simulink model "wheel_leg_robot"  (R2023b)
settings: Solver=ode45  StartTime=0.0  StopTime=10  RelTol=1e-3  AbsTol=1e-3  EnableMultiTasking=on
values from neighbouring files (symbols this model uses):
  N = Nm + mp * (dd_x + L * dd_theta * cos(theta) - L * d_theta^2 * sin(theta))    [model.m]
undefined symbols (not defined in the file or in its folder): X, Y, Z
libraries: sm_lib x57, nesl_utility x19, slpidlib x5, simulink x1
(part 3 of 3)

== matlab function wheel_leg_robot/wheel_leg/MATLAB Function1 ==
  data: phi_1 input; d_phi_1 input; phi_4 input; L0_R output; phi0_R output; d_phi_4 input; d_phi0_R output
function [L0_R, phi0_R, d_phi0_R] = fcn(phi_1, d_phi_1, phi_4, d_phi_4)

    l1 = 0.15;
    l2 = 0.27;
    l3 = l2;
    l4 = l1;
    l5 = 0.15;
    Xb = l1 * cos(phi_1);
    Yb = l1 * sin(phi_1);
    Xd = l4 * cos(phi_4) + l5;
    Yd = l4 * sin(phi_4);
    lbd = sqrt((Xd - Xb)^2 + (Yd - Yb)^2);
    A0 = 2 * l2 * (Xd - Xb);
    B0 = 2 * l2 * (Yd - Yb);
    C0 = l2^2 + lbd^2 - l3^2;
    phi_2 = 2 * atan2((B0 + sqrt(A0^2 + B0^2 - C0^2)), (A0 + C0));
    Xc = Xb + l2 * cos(phi_2);
    Yc = Yb + l2 * sin(phi_2);

    L0_R = sqrt((Xc - l5/2)^2 + Yc^2);
    phi0_R = atan2(Yc, (Xc - l5/2));

    d_phi0_R = (d_phi_1*((l1*cos(phi_1) + (2*l2*cos(2*atan(((4*l2^2*(l1*sin(phi_1) - l4*sin(phi_4))^2 - ((l1*sin(phi_1) - l4*sin(phi_4))^2 + (l5 - l1*cos(phi_1) + l4*cos(phi_4))^2 + l2^2 - l3^2)^2 + 4*l2^2*(l5 - l1*cos(phi_1) + l4*cos(phi_4))^2)^(1/2) - 2*l2*(l1*sin(phi_1) - l4*sin(phi_4)))/((l1*sin(phi_1) - l4*sin(phi_4))^2 + (l5 - l1*cos(phi_1) + l4*cos(phi_4))^2 + l2^2 - l3^2 + 2*l2*(l5 - l1*cos(phi_1) + l4*cos(phi_4)))))*(((8*l1*l2^2*cos(phi_1)*(l1*sin(phi_1) - l4*sin(phi_4)) - 2*(2*l1*cos(phi_1)*(l1*sin(phi_1) - l4*sin(phi_4)) + 2*l1*sin(phi_1)*(l5 - l1*cos(phi_1) + l4*cos(phi_4)))*((l1*sin(phi_1) - l4*sin(phi_4))^2 + (l5 - l1*cos(phi_1) + l4*cos(phi_4))^2 + l2^2 - l3^2) + 8*l1*l2^2*sin(phi_1)*(l5 - l1*cos(phi_1) + l4*cos(phi_4)))/(2*(4*l2^2*(l1*sin(phi_1) - l4*sin(phi_4))^2 - ((l1*sin(phi_1) - l4*sin(phi_4))^2 + (l5 - l1*cos(phi_1) + l4*cos(phi_4))^2 + l2^2 - l3^2)^2 + 4*l2^2*(l5 - l1*cos(phi_1) + l4*cos(phi_4))^2)^(1/2)) - 2*l1*l2*cos(phi_1))/((l1*sin(phi_1) - l4*sin(phi_4))^2 + (l5 - l1*cos(phi_1) + l4*cos(phi_4))^2 + l2^2 - l3^2 + 2*l2*(l5 - l1*cos(phi_1) + l4*cos(phi_4))) - (((4*l2^2*(l1*sin(phi_1) - l4*sin(phi_4))^2 - ((l1*sin(phi_1) - l4*sin(phi_4))^2 + (l5 - l1*cos(phi_1) + l4*cos(phi_4))^2 + l2^2 - l3^2)^2 + 4*l2^2*(l5 - l1*cos(phi_1) + l4*cos(phi_4))^2)^(1/2) - 2*l2*(l1*sin(phi_1) - l4*sin(phi_4)))*(2*l1*l2*sin(phi_1) + 2*l1*cos(phi_1)*(l1*sin(phi_1) - l4*sin(phi_4)) + 2*l1*sin(phi_1)*(l5 - l1*cos(phi_1) + l4*cos(phi_4))))/((l1*sin(phi_1) - l4*sin(phi_4))^2 + (l5 - l1*cos(phi_1) + l4*cos(phi_4))^2 + l2^2 - l3^2 + 2*l2*(l5 - l1*cos(phi_1) + l4*cos(phi_4)))^2))/(((4*l2^2*(l1*sin(phi_1) - l4*sin(phi_4))^2 - ((l1*sin(phi_1) - l4*sin(phi_4))^2 + (l5 - l1*cos(phi_1) + l4*cos(phi_4))^2 + l2^2 - l3^2)^2 + 4*l2^2*(l5 - l1*cos(phi_1) + l4*cos(phi_4))^2)^(1/2) - 2*l2*(l1*sin(phi_1) - l4*sin(phi_4)))^2/((l1*sin(phi_1) - l4*sin(phi_4))^2 + (l5 - l1*cos(phi_1) + l4*cos(phi_4))^2 + l2^2 - l3^2 + 2*l2*(l5 - l1*cos(phi_1) + l4*cos(phi_4)))^2 + 1))/(l2*cos(2*atan(((4*l2^2*(l1*sin(phi_1) - l4*sin(phi_4))^2 - ((l1*sin(phi_1) - l4*sin(phi_4))^2 + (l5 - l1*cos(phi_1) + l4*cos(phi_4))^2 + l2^2 - l3^2)^2 + 4*l2^2*(l5 - l1*cos(phi_1) + l4*cos(phi_4))^2)^(1/2) - 2*l2*(l1*sin(phi_1) - l4*sin(phi_4)))/((l1*sin(phi_1) - l4*sin(phi_4))^2 + (l5 - l1*cos(phi_1) + l4*cos(phi_4))^2 + l2^2 - l3^2 + 2*l2*(l5 - l1*cos(phi_1) + l4*cos(phi_4))))) - l5/2 + l1*cos(phi_1)) + ((l2*sin(2*atan(((4*l2^2*(l1*sin(phi_1) - l4*sin(phi_4))^2 - ((l1*sin(phi_1) - l4*sin(phi_4))^2 + (l5 - l1*cos(phi_1) + l4*cos(phi_4))^2 + l2^2 - l3^2)^2 + 4*l2^2*(l5 - l1*cos(phi_1) + l4*cos(phi_4))^2)^(1/2) - 2*l2*(l1*sin(phi_1) - l4*sin(phi_4)))/((l1*sin(phi_1) - l4*sin(phi_4))^2 + (l5 - l1*cos(phi_1) + l4*cos(phi_4))^2 + l2^2 - l3^2 + 2*l2*(l5 - l1*cos(phi_1) + l4*cos(phi_4))))) + l1*sin(phi_1))*(l1*sin(phi_1) + (2*l2*sin(2*atan(((4*l2^2*(l1*sin(phi_1) - l4*sin(phi_4))^2 - ((l1*sin(phi_1) - l4*sin(phi_4))^2 + (l5 - l1*cos(phi_1) + l4*cos(phi_4))^2 + l2^2 - l3^2)^2 + 4*l2^2*(l5 - l1*cos(phi_1) + l4*cos(phi_4))^2)^(1/2) - 2*l2*(l1*sin(phi_1) - l4*sin(phi_4)))/((l1*sin(phi_1) - l4*sin(phi_4))^2 + (l5 - l1*cos(phi_1) + l4*cos(phi_4))^2 + l2^2 - l3^2 + 2*l2*(l5 - l1*cos(phi_1) + l4*cos(phi_4)))))*(((8*l1*l2^2*cos(phi_1)*(l1*sin(phi_1) - l4*sin(phi_4)) - 2*(2*l1*cos(phi_1)*(l1*sin(phi_1) - l4*sin(phi_4)) + 2*l1*sin(phi_1)*(l5 - l1*cos(phi_1) + l4*cos(phi_4)))*((l1*sin(phi_1) - l4*sin(phi_4))^2 + (l5 - l1*cos(phi_1) + l4*cos(phi_4))^2 + l2^2 - l3^2) + 8*l1*l2^2*sin(phi_1)*(l5 - l1*cos(phi_1) + l4*cos(phi_4)))/(2*(4*l2^2*(l1*sin(phi_1) - l4*sin(phi_4))^2 - ((l1*sin(phi_1) - l4*sin(phi_4))^2 + (l5 - l1*cos(phi_1) + l4*cos(phi_4))^2 + l2^2 - l3^2)^2 + 4*l2^2*(l5 - l1*cos(phi_1) + l4*cos(phi_4))^2)^(1/2)) - 2*l1*l2*cos(phi_1))/((l1*sin(phi_1) - l4*sin(phi_4))^2 + (l5 - l1*cos(phi_1) + l4*cos(phi_4))^2 + l2^2 - l3^2 + 2*l2*(l5 - l1*cos(phi_1) + l4*cos(phi_4))) - (((4*l2^2*(l1*sin(phi_1) - l4*sin(phi_4))^2 - ((l1*sin(phi_1) - l4*sin(phi_4))^2 + (l5 - l1*cos(phi_1) + l4*cos(phi_4))^2 + l2^2 - l3^2)^2 + 4*l2^2*(l5 - l1*cos(phi_1) + l4*cos(phi_4))^2)^(1/2) - 2*l2*(l1*sin(phi_1) - l4*sin(phi_4)))*(2*l1*l2*sin(phi_1) + 2*l1*cos(phi_1)*(l1*sin(phi_1) - l4*sin(phi_4)) + 2*l1*sin(phi_1)*(l5 - l1*cos(phi_1) + l4*cos(phi_4))))/((l1*sin(phi_1) - l4*sin(phi_4))^2 + (l5 - l1*cos(phi_1) + l4*cos(phi_4))^2 + l2^2 - l3^2 + 2*l2*(l5 - l1*cos(phi_1) + l4*cos(phi_4)))^2))/(((4*l2^2*(l1*sin(phi_1) - l4*sin(phi_4))^2 - ((l1*sin(phi_1) - l4*sin(phi_4))^2 + (l5 - l1*cos(phi_1) + l4*cos(phi_4))^2 + l2^2 - l3^2)^2 + 4*l2^2*(l5 - l1*cos(phi_1) + l4*cos(phi_4))^2)^(1/2) - 2*l2*(l1*sin(phi_1) - l4*sin(phi_4)))^2/((l1*sin(phi_1) - l4*sin(phi_4))^2 + (l5 - l1*cos(phi_1) + l4*cos(phi_4))^2 + l2^2 - l3^2 + 2*l2*(l5 - l1*cos(phi_1) + l4*cos(phi_4)))^2 + 1)))/(l2*cos(2*atan(((4*l2^2*(l1*sin(phi_1) - l4*sin(phi_4))^2 - ((l1*sin(phi_1) - l4*sin(phi_4))^2 + (l5 - l1*cos(phi_1) + l4*cos(phi_4))^2 + l2^2 - l3^2)^2 + 4*l2^2*(l5 - l1*cos(phi_1) + l4*cos(phi_4))^2)^(1/2) - 2*l2*(l1*sin(phi_1) - l4*sin(phi_4)))/((l1*sin(phi_1) - l4*sin(phi_4))^2 + (l5 - l1*cos(phi_1) + l4*cos(phi_4))^2 + l2^2 - l3^2 + 2*l2*(l5 - l1*cos(phi_1) + l4*cos(phi_4))))) - l5/2 + l1*cos(phi_1))^2))/((l2*sin(2*atan(((4*l2^2*(l1*sin(phi_1) - l4*sin(phi_4))^2 - ((l1*sin(phi_1) - l4*sin(phi_4))^2 + (l5 - l1*cos(phi_1) + l4*cos(phi_4))^2 + l2^2 - l3^2)^2 + 4*l2^2*(l5 - l1*cos(phi_1) + l4*cos(phi_4))^2)^(1/2) - 2*l2*(l1*sin(phi_1) - l4*sin(phi_4)))/((l1*sin(phi_1) - l4*sin(phi_4))^2 + (l5 - l1*cos(phi_1) + l4*cos(phi_4))^2 + l2^2 - l3^2 + 2*l2*(l5 - l1*cos(phi_1) + l4*cos(phi_4))))) + l1*sin(phi_1))^2/(l2*cos(2*atan(((4*l2^2*(l1*sin(phi_1) - l4*sin(phi_4))^2 - ((l1*sin(phi_1) - l4*sin(phi_4))^2 + (l5 - l1*cos(phi_1) + l4*cos(phi_4))^2 + l2^2 - l3^2)^2 + 4*l2^2*(l5 - l1*cos(phi_1) + l4*cos(phi_4))^2)^(1/2) - 2*l2*(l1*sin(phi_1) - l4*sin(phi_4)))/((l1*sin(phi_1) - l4*sin(phi_4))^2 + (l5 - l1*cos(phi_1) + l4*cos(phi_4))^2 + l2^2 - l3^2 + 2*l2*(l5 - l1*cos(phi_1) + l4*cos(phi_4))))) - l5/2 + l1*cos(phi_1))^2 + 1) - (d_phi_4*((2*l2*cos(2*atan(((4*l2^2*(l1*sin(phi_1) - l4*sin(phi_4))^2 - ((l1*sin(phi_1) - l4*sin(phi_4))^2 + (l5 - l1*cos(phi_1) + l4*cos(phi_4))^2 + l2^2 - l3^2)^2 + 4*l2^2*(l5 - l1*cos(phi_1) + l4*cos(phi_4))^2)^(1/2) - 2*l2*(l1*sin(phi_1) - l4*sin(phi_4)))/((l1*sin(phi_1) - l4*sin(phi_4))^2 + (l5 - l1*cos(phi_1) + l4*cos(phi_4))^2 + l2^2 - l3^2 + 2*l2*(l5 - l1*cos(phi_1) + l4*cos(phi_4)))))*(((8*l2^2*l4*cos(phi_4)*(l1*sin(phi_1) - l4*sin(phi_4)) - 2*(2*l4*cos(phi_4)*(l1*sin(phi_1) - l4*sin(phi_4)) + 2*l4*sin(phi_4)*(l5 - l1*cos(phi_1) + l4*cos(phi_4)))*((l1*sin(phi_1) - l4*sin(phi_4))^2 + (l5 - l1*cos(phi_1) + l4*cos(phi_4))^2 + l2^2 - l3^2) + 8*l2^2*l4*sin(phi_4)*(l5 - l1*cos(phi_1) + l4*cos(phi_4)))/(2*(4*l2^2*(l1*sin(phi_1) - l4*sin(phi_4))^2 - ((l1*sin(phi_1) - l4*sin(phi_4))^2 + (l5 - l1*cos(phi_1) + l4*cos(phi_4))^2 + l2^2 - l3^2)^2 + 4*l2^2*(l5 - l1*cos(phi_1) + l4*cos(phi_4))^2)^(1/2)) - 2*l2*l4*cos(phi_4))/((l1*sin(phi_1) - l4*sin(phi_4))^2 + (l5 - l1*cos(phi_1) + l4*cos(phi_4))^2 + l2^2 - l3^2 + 2*l2*(l5 - l1*cos(phi_1) + l4*cos(phi_4))) - (((4*l2^2*(l1*sin(phi_1) - l4*sin(phi_4))^2 - ((l1*sin(phi_1) - l4*sin(phi_4))^2 + (l5 - l1*cos(phi_1) + l4*cos(phi_4))^2 + l2^2 - l3^2)^2 + 4*l2^2*(l5 - l1*cos(phi_1) + l4*cos(phi_4))^2)^(1/2) - 2*l2*(l1*sin(phi_1) - l4*sin(phi_4)))*(2*l2*l4*sin(phi_4) + 2*l4*cos(phi_4)*(l1*sin(phi_1) - l4*sin(phi_4)) + 2*l4*sin(phi_4)*(l5 - l1*cos(phi_1) + l4*cos(phi_4))))/((l1*sin(phi_1) - l4*sin(phi_4))^2 + (l5 - l1*cos(phi_1) + l4*cos(phi_4))^2 + l2^2 - l3^2 + 2*l2*(l5 - l1*cos(phi_1) + l4*cos(phi_4)))^2))/((((4*l2^2*(l1*sin(phi_1) - l4*sin(phi_4))^2 - ((l1*sin(phi_1) - l4*sin(phi_4))^2 + (l5 - l1*cos(phi_1) + l4*cos(phi_4))^2 + l2^2 - l3^2)^2 + 4*l2^2*(l5 - l1*cos(phi_1) + l4*cos(phi_4))^2)^(1/2) - 2*l2*(l1*sin(phi_1) - l4*sin(phi_4)))^2/((l1*sin(phi_1) - l4*sin(phi_4))^2 + (l5 - l1*cos(phi_1) + l4*cos(phi_4))^2 + l2^2 - l3^2 + 2*l2*(l5 - l1*cos(phi_1) + l4*cos(phi_4)))^2 + 1)*(l2*cos(2*atan(((4*l2^2*(l1*sin(phi_1) - l4*sin(phi_4))^2 - ((l1*sin(phi_1) - l4*sin(phi_4))^2 + (l5 - l1*cos(phi_1) + l4*cos(phi_4))^2 + l2^2 - l3^2)^2 + 4*l2^2*(l5 - l1*cos(phi_1) + l4*cos(phi_4))^2)^(1/2) - 2*l2*(l1*sin(phi_1) - l4*sin(phi_4)))/((l1*sin(phi_1) - l4*sin(phi_4))^2 + (l5 - l1*cos(phi_1) + l4*cos(phi_4))^2 + l2^2 - l3^2 + 2*l2*(l5 - l1*cos(phi_1) + l4*cos(phi_4))))) - l5/2 + l1*cos(phi_1))) + (2*l2*sin(2*atan(((4*l2^2*(l1*sin(phi_1) - l4*sin(phi_4))^2 - ((l1*sin(phi_1) - l4*sin(phi_4))^2 + (l5 - l1*cos(phi_1) + l4*cos(phi_4))^2 + l2^2 - l3^2)^2 + 4*l2^2*(l5 - l1*cos(phi_1) + l4*cos(phi_4))^2)^(1/2) - 2*l2*(l1*sin(phi_1) - l4*sin(phi_4)))/((l1*sin(phi_1) - l4*sin(phi_4))^2 + (l5 - l1*cos(phi_1) + l4*cos(phi_4))^2 + l2^2 - l3^2 + 2*l2*(l5 - l1*cos(phi_1) + l4*cos(phi_4)))))*(l2*sin(2*atan(((4*l2^2*(l1*sin(phi_1) - l4*sin(phi_4))^2 - ((l1*sin(phi_1) - l4*sin(phi_4))^2 + (l5 - l1*cos(phi_1) + l4*cos(phi_4))^2 + l2^2 - l3^2)^2 + 4*l2^2*(l5 - l1*cos(phi_1) + l4*cos(phi_4))^2)^(1/2) - 2*l2*(l1*sin(phi_1) - l4*sin(phi_4)))/((l1*sin(phi_1) - l4*sin(phi_4))^2 + (l5 - l1*cos(phi_1) + l4*cos(phi_4))^2 + l2^2 - l3^2 + 2*l2*(l5 - l1*cos(phi_1) + l4*cos(phi_4))))) + l1*sin(phi_1))*(((8*l2^2*l4*cos(phi_4)*(l1*sin(phi_1) - l4*sin(phi_4)) - 2*(2*l4*cos(phi_4)*(l1*sin(phi_1) - l4*sin(phi_4)) + 2*l4*sin(phi_4)*(l5 - l1*cos(phi_1) + l4*cos(phi_4)))*((l1*sin(phi_1) - l4*sin(phi_4))^2 + (l5 - l1*cos(phi_1) + l4*cos(phi_4))^2 + l2^2 - l3^2) + 8*l2^2*l4*sin(phi_4)*(l5 - l1*cos(phi_1) + l4*cos(phi_4)))/(2*(4*l2^2*(l1*sin(phi_1) - l4*sin(phi_4))^2 - ((l1*sin(phi_1) - l4*sin(phi_4))^2 + (l5 - l1*cos(phi_1) + l4*cos(phi_4))^2 + l2^2 - l3^2)^2 + 4*l2^2*(l5 - l1*cos(phi_1) + l4*cos(phi_4))^2)^(1/2)) - 2*l2*l4*cos(phi_4))/((l1*sin(phi_1) - l4*sin(phi_4))^2 + (l5 - l1*cos(phi_1) + l4*cos(phi_4))^2 + l2^2 - l3^2 + 2*l2*(l5 - l1*cos(phi_1) + l4*cos(phi_4))) - (((4*l2^2*(l1*sin(phi_1) - l4*sin(phi_4))^2 - ((l1*sin(phi_1) - l4*sin(phi_4))^2 + (l5 - l1*cos(phi_1) + l4*cos(phi_4))^2 + l2^2 - l3^2)^2 + 4*l2^2*(l5 - l1*cos(phi_1) + l4*cos(phi_4))^2)^(1/2) - 2*l2*(l1*sin(phi_1) - l4*sin(phi_4)))*(2*l2*l4*sin(phi_4) + 2*l4*cos(phi_4)*(l1*sin(phi_1) - l4*sin(phi_4)) + 2*l4*sin(phi_4)*(l5 - l1*cos(phi_1) + l4*cos(phi_4))))/((l1*sin(phi_1) - l4*sin(phi_4))^2 + (l5 - l1*cos(phi_1) + l4*cos(phi_4))^2 + l2^2 - l3^2 + 2*l2*(l5 - l1*cos(phi_1) + l4*cos(phi_4)))^2))/((((4*l2^2*(l1*sin(phi_1) - l4*sin(phi_4))^2 - ((l1*sin(phi_1) - l4*sin(phi_4))^2 + (l5 - l1*cos(phi_1) + l4*cos(phi_4))^2 + l2^2 - l3^2)^2 + 4*l2^2*(l5 - l1*cos(phi_1) + l4*cos(phi_4))^2)^(1/2) - 2*l2*(l1*sin(phi_1) - l4*sin(phi_4)))^2/((l1*sin(phi_1) - l4*sin(phi_4))^2 + (l5 - l1*cos(phi_1) + l4*cos(phi_4))^2 + l2^2 - l3^2 + 2*l2*(l5 - l1*cos(phi_1) + l4*cos(phi_4)))^2 + 1)*(l2*cos(2*atan(((4*l2^2*(l1*sin(phi_1) - l4*sin(phi_4))^2 - ((l1*sin(phi_1) - l4*sin(phi_4))^2 + (l5 - l1*cos(phi_1) + l4*cos(phi_4))^2 + l2^2 - l3^2)^2 + 4*l2^2*(l5 - l1*cos(phi_1) + l4*cos(phi_4))^2)^(1/2) - 2*l2*(l1*sin(phi_1) - l4*sin(phi_4)))/((l1*sin(phi_1) - l4*sin(phi_4))^2 + (l5 - l1*cos(phi_1) + l4*cos(phi_4))^2 + l2^2 - l3^2 + 2*l2*(l5 - l1*cos(phi_1) + l4*cos(phi_4))))) - l5/2 + l1*cos(phi_1))^2)))/((l2*sin(2*atan(((4*l2^2*(l1*sin(phi_1) - l4*sin(phi_4))^2 - ((l1*sin(phi_1) - l4*sin(phi_4))^2 + (l5 - l1*cos(phi_1) + l4*cos(phi_4))^2 + l2^2 - l3^2)^2 + 4*l2^2*(l5 - l1*cos(phi_1) + l4*cos(phi_4))^2)^(1/2) - 2*l2*(l1*sin(phi_1) - l4*sin(phi_4)))/((l1*sin(phi_1) - l4*sin(phi_4))^2 + (l5 - l1*cos(phi_1) + l4*cos(phi_4))^2 + l2^2 - l3^2 + 2*l2*(l5 - l1*cos(phi_1) + l4*cos(phi_4))))) + l1*sin(phi_1))^2/(l2*cos(2*atan(((4*l2^2*(l1*sin(phi_1) - l4*sin(phi_4))^2 - ((l1*sin(phi_1) - l4*sin(phi_4))^2 + (l5 - l1*cos(phi_1) + l4*cos(phi_4))^2 + l2^2 - l3^2)^2 + 4*l2^2*(l5 - l1*cos(phi_1) + l4*cos(phi_4))^2)^(1/2) - 2*l2*(l1*sin(phi_1) - l4*sin(phi_4)))/((l1*sin(phi_1) - l4*sin(phi_4))^2 + (l5 - l1*cos(phi_1) + l4*cos(phi_4))^2 + l2^2 - l3^2 + 2*l2*(l5 - l1*cos(phi_1) + l4*cos(phi_4))))) - l5/2 + l1*cos(phi_1))^2 + 1);

== matlab function wheel_leg_robot/wheel_leg/MATLAB Function ==
  data: phi_1 input; d_phi_1 input; phi_4 input; L0_L output; phi0_L output; d_phi_4 input; d_phi0_L output
function [L0_L, phi0_L, d_phi0_L] = fcn(phi_1, d_phi_1, phi_4, d_phi_4)

    l1 = 0.15;
    l2 = 0.27;
    l3 = l2;
    l4 = l1;
    l5 = 0.15;
    Xb = l1 * cos(phi_1);
    Yb = l1 * sin(phi_1);
    Xd = l4 * cos(phi_4) + l5;
    Yd = l4 * sin(phi_4);
    lbd = sqrt((Xd - Xb)^2 + (Yd - Yb)^2);
    A0 = 2 * l2 * (Xd - Xb);
    B0 = 2 * l2 * (Yd - Yb);
    C0 = l2^2 + lbd^2 - l3^2;
    phi_2 = 2 * atan2((B0 + sqrt(A0^2 + B0^2 - C0^2)), (A0 + C0));
    Xc = Xb + l2 * cos(phi_2);
    Yc = Yb + l2 * sin(phi_2);

    L0_L = sqrt((Xc - l5/2)^2 + Yc^2);
    phi0_L = atan2(Yc, (Xc - l5/2));

    d_phi0_L = (d_phi_1*((l1*cos(phi_1) + (2*l2*cos(2*atan(((4*l2^2*(l1*sin(phi_1) - l4*sin(phi_4))^2 - ((l1*sin(phi_1) - l4*sin(phi_4))^2 + (l5 - l1*cos(phi_1) + l4*cos(phi_4))^2 + l2^2 - l3^2)^2 + 4*l2^2*(l5 - l1*cos(phi_1) + l4*cos(phi_4))^2)^(1/2) - 2*l2*(l1*sin(phi_1) - l4*sin(phi_4)))/((l1*sin(phi_1) - l4*sin(phi_4))^2 + (l5 - l1*cos(phi_1) + l4*cos(phi_4))^2 + l2^2 - l3^2 + 2*l2*(l5 - l1*cos(phi_1) + l4*cos(phi_4)))))*(((8*l1*l2^2*cos(phi_1)*(l1*sin(phi_1) - l4*sin(phi_4)) - 2*(2*l1*cos(phi_1)*(l1*sin(phi_1) - l4*sin(phi_4)) + 2*l1*sin(phi_1)*(l5 - l1*cos(phi_1) + l4*cos(phi_4)))*((l1*sin(phi_1) - l4*sin(phi_4))^2 + (l5 - l1*cos(phi_1) + l4*cos(phi_4))^2 + l2^2 - l3^2) + 8*l1*l2^2*sin(phi_1)*(l5 - l1*cos(phi_1) + l4*cos(phi_4)))/(2*(4*l2^2*(l1*sin(phi_1) - l4*sin(phi_4))^2 - ((l1*sin(phi_1) - l4*sin(phi_4))^2 + (l5 - l1*cos(phi_1) + l4*cos(phi_4))^2 + l2^2 - l3^2)^2 + 4*l2^2*(l5 - l1*cos(phi_1) + l4*cos(phi_4))^2)^(1/2)) - 2*l1*l2*cos(phi_1))/((l1*sin(phi_1) - l4*sin(phi_4))^2 + (l5 - l1*cos(phi_1) + l4*cos(phi_4))^2 + l2^2 - l3^2 + 2*l2*(l5 - l1*cos(phi_1) + l4*cos(phi_4))) - (((4*l2^2*(l1*sin(phi_1) - l4*sin(phi_4))^2 - ((l1*sin(phi_1) - l4*sin(phi_4))^2 + (l5 - l1*cos(phi_1) + l4*cos(phi_4))^2 + l2^2 - l3^2)^2 + 4*l2^2*(l5 - l1*cos(phi_1) + l4*cos(phi_4))^2)^(1/2) - 2*l2*(l1*sin(phi_1) - l4*sin(phi_4)))*(2*l1*l2*sin(phi_1) + 2*l1*cos(phi_1)*(l1*sin(phi_1) - l4*sin(phi_4)) + 2*l1*sin(phi_1)*(l5 - l1*cos(phi_1) + l4*cos(phi_4))))/((l1*sin(phi_1) - l4*sin(phi_4))^2 + (l5 - l1*cos(phi_1) + l4*cos(phi_4))^2 + l2^2 - l3^2 + 2*l2*(l5 - l1*cos(phi_1) + l4*cos(phi_4)))^2))/(((4*l2^2*(l1*sin(phi_1) - l4*sin(phi_4))^2 - ((l1*sin(phi_1) - l4*sin(phi_4))^2 + (l5 - l1*cos(phi_1) + l4*cos(phi_4))^2 + l2^2 - l3^2)^2 + 4*l2^2*(l5 - l1*cos(phi_1) + l4*cos(phi_4))^2)^(1/2) - 2*l2*(l1*sin(phi_1) - l4*sin(phi_4)))^2/((l1*sin(phi_1) - l4*sin(phi_4))^2 + (l5 - l1*cos(phi_1) + l4*cos(phi_4))^2 + l2^2 - l3^2 + 2*l2*(l5 - l1*cos(phi_1) + l4*cos(phi_4)))^2 + 1))/(l2*cos(2*atan(((4*l2^2*(l1*sin(phi_1) - l4*sin(phi_4))^2 - ((l1*sin(phi_1) - l4*sin(phi_4))^2 + (l5 - l1*cos(phi_1) + l4*cos(phi_4))^2 + l2^2 - l3^2)^2 + 4*l2^2*(l5 - l1*cos(phi_1) + l4*cos(phi_4))^2)^(1/2) - 2*l2*(l1*sin(phi_1) - l4*sin(phi_4)))/((l1*sin(phi_1) - l4*sin(phi_4))^2 + (l5 - l1*cos(phi_1) + l4*cos(phi_4))^2 + l2^2 - l3^2 + 2*l2*(l5 - l1*cos(phi_1) + l4*cos(phi_4))))) - l5/2 + l1*cos(phi_1)) + ((l2*sin(2*atan(((4*l2^2*(l1*sin(phi_1) - l4*sin(phi_4))^2 - ((l1*sin(phi_1) - l4*sin(phi_4))^2 + (l5 - l1*cos(phi_1) + l4*cos(phi_4))^2 + l2^2 - l3^2)^2 + 4*l2^2*(l5 - l1*cos(phi_1) + l4*cos(phi_4))^2)^(1/2) - 2*l2*(l1*sin(phi_1) - l4*sin(phi_4)))/((l1*sin(phi_1) - l4*sin(phi_4))^2 + (l5 - l1*cos(phi_1) + l4*cos(phi_4))^2 + l2^2 - l3^2 + 2*l2*(l5 - l1*cos(phi_1) + l4*cos(phi_4))))) + l1*sin(phi_1))*(l1*sin(phi_1) + (2*l2*sin(2*atan(((4*l2^2*(l1*sin(phi_1) - l4*sin(phi_4))^2 - ((l1*sin(phi_1) - l4*sin(phi_4))^2 + (l5 - l1*cos(phi_1) + l4*cos(phi_4))^2 + l2^2 - l3^2)^2 + 4*l2^2*(l5 - l1*cos(phi_1) + l4*cos(phi_4))^2)^(1/2) - 2*l2*(l1*sin(phi_1) - l4*sin(phi_4)))/((l1*sin(phi_1) - l4*sin(phi_4))^2 + (l5 - l1*cos(phi_1) + l4*cos(phi_4))^2 + l2^2 - l3^2 + 2*l2*(l5 - l1*cos(phi_1) + l4*cos(phi_4)))))*(((8*l1*l2^2*cos(phi_1)*(l1*sin(phi_1) - l4*sin(phi_4)) - 2*(2*l1*cos(phi_1)*(l1*sin(phi_1) - l4*sin(phi_4)) + 2*l1*sin(phi_1)*(l5 - l1*cos(phi_1) + l4*cos(phi_4)))*((l1*sin(phi_1) - l4*sin(phi_4))^2 + (l5 - l1*cos(phi_1) + l4*cos(phi_4))^2 + l2^2 - l3^2) + 8*l1*l2^2*sin(phi_1)*(l5 - l1*cos(phi_1) + l4*cos(phi_4)))/(2*(4*l2^2*(l1*sin(phi_1) - l4*sin(phi_4))^2 - ((l1*sin(phi_1) - l4*sin(phi_4))^2 + (l5 - l1*cos(phi_1) + l4*cos(phi_4))^2 + l2^2 - l3^2)^2 + 4*l2^2*(l5 - l1*cos(phi_1) + l4*cos(phi_4))^2)^(1/2)) - 2*l1*l2*cos(phi_1))/((l1*sin(phi_1) - l4*sin(phi_4))^2 + (l5 - l1*cos(phi_1) + l4*cos(phi_4))^2 + l2^2 - l3^2 + 2*l2*(l5 - l1*cos(phi_1) + l4*cos(phi_4))) - (((4*l2^2*(l1*sin(phi_1) - l4*sin(phi_4))^2 - ((l1*sin(phi_1) - l4*sin(phi_4))^2 + (l5 - l1*cos(phi_1) + l4*cos(phi_4))^2 + l2^2 - l3^2)^2 + 4*l2^2*(l5 - l1*cos(phi_1) + l4*cos(phi_4))^2)^(1/2) - 2*l2*(l1*sin(phi_1) - l4*sin(phi_4)))*(2*l1*l2*sin(phi_1) + 2*l1*cos(phi_1)*(l1*sin(phi_1) - l4*sin(phi_4)) + 2*l1*sin(phi_1)*(l5 - l1*cos(phi_1) + l4*cos(phi_4))))/((l1*sin(phi_1) - l4*sin(phi_4))^2 + (l5 - l1*cos(phi_1) + l4*cos(phi_4))^2 + l2^2 - l3^2 + 2*l2*(l5 - l1*cos(phi_1) + l4*cos(phi_4)))^2))/(((4*l2^2*(l1*sin(phi_1) - l4*sin(phi_4))^2 - ((l1*sin(phi_1) - l4*sin(phi_4))^2 + (l5 - l1*cos(phi_1) + l4*cos(phi_4))^2 + l2^2 - l3^2)^2 + 4*l2^2*(l5 - l1*cos(phi_1) + l4*cos(phi_4))^2)^(1/2) - 2*l2*(l1*sin(phi_1) - l4*sin(phi_4)))^2/((l1*sin(phi_1) - l4*sin(phi_4))^2 + (l5 - l1*cos(phi_1) + l4*cos(phi_4))^2 + l2^2 - l3^2 + 2*l2*(l5 - l1*cos(phi_1) + l4*cos(phi_4)))^2 + 1)))/(l2*cos(2*atan(((4*l2^2*(l1*sin(phi_1) - l4*sin(phi_4))^2 - ((l1*sin(phi_1) - l4*sin(phi_4))^2 + (l5 - l1*cos(phi_1) + l4*cos(phi_4))^2 + l2^2 - l3^2)^2 + 4*l2^2*(l5 - l1*cos(phi_1) + l4*cos(phi_4))^2)^(1/2) - 2*l2*(l1*sin(phi_1) - l4*sin(phi_4)))/((l1*sin(phi_1) - l4*sin(phi_4))^2 + (l5 - l1*cos(phi_1) + l4*cos(phi_4))^2 + l2^2 - l3^2 + 2*l2*(l5 - l1*cos(phi_1) + l4*cos(phi_4))))) - l5/2 + l1*cos(phi_1))^2))/((l2*sin(2*atan(((4*l2^2*(l1*sin(phi_1) - l4*sin(phi_4))^2 - ((l1*sin(phi_1) - l4*sin(phi_4))^2 + (l5 - l1*cos(phi_1) + l4*cos(phi_4))^2 + l2^2 - l3^2)^2 + 4*l2^2*(l5 - l1*cos(phi_1) + l4*cos(phi_4))^2)^(1/2) - 2*l2*(l1*sin(phi_1) - l4*sin(phi_4)))/((l1*sin(phi_1) - l4*sin(phi_4))^2 + (l5 - l1*cos(phi_1) + l4*cos(phi_4))^2 + l2^2 - l3^2 + 2*l2*(l5 - l1*cos(phi_1) + l4*cos(phi_4))))) + l1*sin(phi_1))^2/(l2*cos(2*atan(((4*l2^2*(l1*sin(phi_1) - l4*sin(phi_4))^2 - ((l1*sin(phi_1) - l4*sin(phi_4))^2 + (l5 - l1*cos(phi_1) + l4*cos(phi_4))^2 + l2^2 - l3^2)^2 + 4*l2^2*(l5 - l1*cos(phi_1) + l4*cos(phi_4))^2)^(1/2) - 2*l2*(l1*sin(phi_1) - l4*sin(phi_4)))/((l1*sin(phi_1) - l4*sin(phi_4))^2 + (l5 - l1*cos(phi_1) + l4*cos(phi_4))^2 + l2^2 - l3^2 + 2*l2*(l5 - l1*cos(phi_1) + l4*cos(phi_4))))) - l5/2 + l1*cos(phi_1))^2 + 1) - (d_phi_4*((2*l2*cos(2*atan(((4*l2^2*(l1*sin(phi_1) - l4*sin(phi_4))^2 - ((l1*sin(phi_1) - l4*sin(phi_4))^2 + (l5 - l1*cos(phi_1) + l4*cos(phi_4))^2 + l2^2 - l3^2)^2 + 4*l2^2*(l5 - l1*cos(phi_1) + l4*cos(phi_4))^2)^(1/2) - 2*l2*(l1*sin(phi_1) - l4*sin(phi_4)))/((l1*sin(phi_1) - l4*sin(phi_4))^2 + (l5 - l1*cos(phi_1) + l4*cos(phi_4))^2 + l2^2 - l3^2 + 2*l2*(l5 - l1*cos(phi_1) + l4*cos(phi_4)))))*(((8*l2^2*l4*cos(phi_4)*(l1*sin(phi_1) - l4*sin(phi_4)) - 2*(2*l4*cos(phi_4)*(l1*sin(phi_1) - l4*sin(phi_4)) + 2*l4*sin(phi_4)*(l5 - l1*cos(phi_1) + l4*cos(phi_4)))*((l1*sin(phi_1) - l4*sin(phi_4))^2 + (l5 - l1*cos(phi_1) + l4*cos(phi_4))^2 + l2^2 - l3^2) + 8*l2^2*l4*sin(phi_4)*(l5 - l1*cos(phi_1) + l4*cos(phi_4)))/(2*(4*l2^2*(l1*sin(phi_1) - l4*sin(phi_4))^2 - ((l1*sin(phi_1) - l4*sin(phi_4))^2 + (l5 - l1*cos(phi_1) + l4*cos(phi_4))^2 + l2^2 - l3^2)^2 + 4*l2^2*(l5 - l1*cos(phi_1) + l4*cos(phi_4))^2)^(1/2)) - 2*l2*l4*cos(phi_4))/((l1*sin(phi_1) - l4*sin(phi_4))^2 + (l5 - l1*cos(phi_1) + l4*cos(phi_4))^2 + l2^2 - l3^2 + 2*l2*(l5 - l1*cos(phi_1) + l4*cos(phi_4))) - (((4*l2^2*(l1*sin(phi_1) - l4*sin(phi_4))^2 - ((l1*sin(phi_1) - l4*sin(phi_4))^2 + (l5 - l1*cos(phi_1) + l4*cos(phi_4))^2 + l2^2 - l3^2)^2 + 4*l2^2*(l5 - l1*cos(phi_1) + l4*cos(phi_4))^2)^(1/2) - 2*l2*(l1*sin(phi_1) - l4*sin(phi_4)))*(2*l2*l4*sin(phi_4) + 2*l4*cos(phi_4)*(l1*sin(phi_1) - l4*sin(phi_4)) + 2*l4*sin(phi_4)*(l5 - l1*cos(phi_1) + l4*cos(phi_4))))/((l1*sin(phi_1) - l4*sin(phi_4))^2 + (l5 - l1*cos(phi_1) + l4*cos(phi_4))^2 + l2^2 - l3^2 + 2*l2*(l5 - l1*cos(phi_1) + l4*cos(phi_4)))^2))/((((4*l2^2*(l1*sin(phi_1) - l4*sin(phi_4))^2 - ((l1*sin(phi_1) - l4*sin(phi_4))^2 + (l5 - l1*cos(phi_1) + l4*cos(phi_4))^2 + l2^2 - l3^2)^2 + 4*l2^2*(l5 - l1*cos(phi_1) + l4*cos(phi_4))^2)^(1/2) - 2*l2*(l1*sin(phi_1) - l4*sin(phi_4)))^2/((l1*sin(phi_1) - l4*sin(phi_4))^2 + (l5 - l1*cos(phi_1) + l4*cos(phi_4))^2 + l2^2 - l3^2 + 2*l2*(l5 - l1*cos(phi_1) + l4*cos(phi_4)))^2 + 1)*(l2*cos(2*atan(((4*l2^2*(l1*sin(phi_1) - l4*sin(phi_4))^2 - ((l1*sin(phi_1) - l4*sin(phi_4))^2 + (l5 - l1*cos(phi_1) + l4*cos(phi_4))^2 + l2^2 - l3^2)^2 + 4*l2^2*(l5 - l1*cos(phi_1) + l4*cos(phi_4))^2)^(1/2) - 2*l2*(l1*sin(phi_1) - l4*sin(phi_4)))/((l1*sin(phi_1) - l4*sin(phi_4))^2 + (l5 - l1*cos(phi_1) + l4*cos(phi_4))^2 + l2^2 - l3^2 + 2*l2*(l5 - l1*cos(phi_1) + l4*cos(phi_4))))) - l5/2 + l1*cos(phi_1))) + (2*l2*sin(2*atan(((4*l2^2*(l1*sin(phi_1) - l4*sin(phi_4))^2 - ((l1*sin(phi_1) - l4*sin(phi_4))^2 + (l5 - l1*cos(phi_1) + l4*cos(phi_4))^2 + l2^2 - l3^2)^2 + 4*l2^2*(l5 - l1*cos(phi_1) + l4*cos(phi_4))^2)^(1/2) - 2*l2*(l1*sin(phi_1) - l4*sin(phi_4)))/((l1*sin(phi_1) - l4*sin(phi_4))^2 + (l5 - l1*cos(phi_1) + l4*cos(phi_4))^2 + l2^2 - l3^2 + 2*l2*(l5 - l1*cos(phi_1) + l4*cos(phi_4)))))*(l2*sin(2*atan(((4*l2^2*(l1*sin(phi_1) - l4*sin(phi_4))^2 - ((l1*sin(phi_1) - l4*sin(phi_4))^2 + (l5 - l1*cos(phi_1) + l4*cos(phi_4))^2 + l2^2 - l3^2)^2 + 4*l2^2*(l5 - l1*cos(phi_1) + l4*cos(phi_4))^2)^(1/2) - 2*l2*(l1*sin(phi_1) - l4*sin(phi_4)))/((l1*sin(phi_1) - l4*sin(phi_4))^2 + (l5 - l1*cos(phi_1) + l4*cos(phi_4))^2 + l2^2 - l3^2 + 2*l2*(l5 - l1*cos(phi_1) + l4*cos(phi_4))))) + l1*sin(phi_1))*(((8*l2^2*l4*cos(phi_4)*(l1*sin(phi_1) - l4*sin(phi_4)) - 2*(2*l4*cos(phi_4)*(l1*sin(phi_1) - l4*sin(phi_4)) + 2*l4*sin(phi_4)*(l5 - l1*cos(phi_1) + l4*cos(phi_4)))*((l1*sin(phi_1) - l4*sin(phi_4))^2 + (l5 - l1*cos(phi_1) + l4*cos(phi_4))^2 + l2^2 - l3^2) + 8*l2^2*l4*sin(phi_4)*(l5 - l1*cos(phi_1) + l4*cos(phi_4)))/(2*(4*l2^2*(l1*sin(phi_1) - l4*sin(phi_4))^2 - ((l1*sin(phi_1) - l4*sin(phi_4))^2 + (l5 - l1*cos(phi_1) + l4*cos(phi_4))^2 + l2^2 - l3^2)^2 + 4*l2^2*(l5 - l1*cos(phi_1) + l4*cos(phi_4))^2)^(1/2)) - 2*l2*l4*cos(phi_4))/((l1*sin(phi_1) - l4*sin(phi_4))^2 + (l5 - l1*cos(phi_1) + l4*cos(phi_4))^2 + l2^2 - l3^2 + 2*l2*(l5 - l1*cos(phi_1) + l4*cos(phi_4))) - (((4*l2^2*(l1*sin(phi_1) - l4*sin(phi_4))^2 - ((l1*sin(phi_1) - l4*sin(phi_4))^2 + (l5 - l1*cos(phi_1) + l4*cos(phi_4))^2 + l2^2 - l3^2)^2 + 4*l2^2*(l5 - l1*cos(phi_1) + l4*cos(phi_4))^2)^(1/2) - 2*l2*(l1*sin(phi_1) - l4*sin(phi_4)))*(2*l2*l4*sin(phi_4) + 2*l4*cos(phi_4)*(l1*sin(phi_1) - l4*sin(phi_4)) + 2*l4*sin(phi_4)*(l5 - l1*cos(phi_1) + l4*cos(phi_4))))/((l1*sin(phi_1) - l4*sin(phi_4))^2 + (l5 - l1*cos(phi_1) + l4*cos(phi_4))^2 + l2^2 - l3^2 + 2*l2*(l5 - l1*cos(phi_1) + l4*cos(phi_4)))^2))/((((4*l2^2*(l1*sin(phi_1) - l4*sin(phi_4))^2 - ((l1*sin(phi_1) - l4*sin(phi_4))^2 + (l5 - l1*cos(phi_1) + l4*cos(phi_4))^2 + l2^2 - l3^2)^2 + 4*l2^2*(l5 - l1*cos(phi_1) + l4*cos(phi_4))^2)^(1/2) - 2*l2*(l1*sin(phi_1) - l4*sin(phi_4)))^2/((l1*sin(phi_1) - l4*sin(phi_4))^2 + (l5 - l1*cos(phi_1) + l4*cos(phi_4))^2 + l2^2 - l3^2 + 2*l2*(l5 - l1*cos(phi_1) + l4*cos(phi_4)))^2 + 1)*(l2*cos(2*atan(((4*l2^2*(l1*sin(phi_1) - l4*sin(phi_4))^2 - ((l1*sin(phi_1) - l4*sin(phi_4))^2 + (l5 - l1*cos(phi_1) + l4*cos(phi_4))^2 + l2^2 - l3^2)^2 + 4*l2^2*(l5 - l1*cos(phi_1) + l4*cos(phi_4))^2)^(1/2) - 2*l2*(l1*sin(phi_1) - l4*sin(phi_4)))/((l1*sin(phi_1) - l4*sin(phi_4))^2 + (l5 - l1*cos(phi_1) + l4*cos(phi_4))^2 + l2^2 - l3^2 + 2*l2*(l5 - l1*cos(phi_1) + l4*cos(phi_4))))) - l5/2 + l1*cos(phi_1))^2)))/((l2*sin(2*atan(((4*l2^2*(l1*sin(phi_1) - l4*sin(phi_4))^2 - ((l1*sin(phi_1) - l4*sin(phi_4))^2 + (l5 - l1*cos(phi_1) + l4*cos(phi_4))^2 + l2^2 - l3^2)^2 + 4*l2^2*(l5 - l1*cos(phi_1) + l4*cos(phi_4))^2)^(1/2) - 2*l2*(l1*sin(phi_1) - l4*sin(phi_4)))/((l1*sin(phi_1) - l4*sin(phi_4))^2 + (l5 - l1*cos(phi_1) + l4*cos(phi_4))^2 + l2^2 - l3^2 + 2*l2*(l5 - l1*cos(phi_1) + l4*cos(phi_4))))) + l1*sin(phi_1))^2/(l2*cos(2*atan(((4*l2^2*(l1*sin(phi_1) - l4*sin(phi_4))^2 - ((l1*sin(phi_1) - l4*sin(phi_4))^2 + (l5 - l1*cos(phi_1) + l4*cos(phi_4))^2 + l2^2 - l3^2)^2 + 4*l2^2*(l5 - l1*cos(phi_1) + l4*cos(phi_4))^2)^(1/2) - 2*l2*(l1*sin(phi_1) - l4*sin(phi_4)))/((l1*sin(phi_1) - l4*sin(phi_4))^2 + (l5 - l1*cos(phi_1) + l4*cos(phi_4))^2 + l2^2 - l3^2 + 2*l2*(l5 - l1*cos(phi_1) + l4*cos(phi_4))))) - l5/2 + l1*cos(phi_1))^2 + 1);

== matlab function wheel_leg_robot/wheel_leg/MATLAB Function2 ==
  data: L0_L input; k_lqr_L output
function k_lqr_L = fcn(L0_L)

k_lqr_L = K_lqr(L0_L);

== matlab function wheel_leg_robot/wheel_leg/MATLAB Function3 ==
  data: L0_R input; k_lqr_R output
function k_lqr_R = fcn(L0_R)

k_lqr_R = K_lqr(L0_R);

== matlab function wheel_leg_robot/wheel_leg/MATLAB Function4 ==
  data: F input; T1_L output; Tp input; phi1 input; phi4 input; T2_L output
function [T1_L, T2_L] = fcn(F, Tp, phi1, phi4)

    l1 = 0.15;
    l2 = 0.27;
    l3 = l2;
    l4 = l1;
    l5 = 0.15;
    Xb = l1 * cos(phi1);
    Yb = l1 * sin(phi1);
    Xd = l4 * cos(phi4) + l5;
    Yd = l4 * sin(phi4);
    lbd = sqrt((Xd - Xb)^2 + (Yd - Yb)^2);
    A0 = 2 * l2 * (Xd - Xb);
    B0 = 2 * l2 * (Yd - Yb);
    C0 = l2^2 + lbd^2 - l3^2;
    phi2 = 2 * atan2((B0 + sqrt(A0^2 + B0^2 - C0^2)), (A0 + C0));
    phi3 = atan2(Yb - Yd + l2 * sin(phi2), Xb - Xd + l2 * cos(phi2));
    Xc = Xb + l2 * cos(phi2);
    Yc = Yb + l2 * sin(phi2);
    l0 = sqrt((Xc - l5/2)^2 + Yc^2);
    phi0 = atan2(Yc, (Xc - l5/2));
    j11 = (l1 * sin(phi0 - phi3) * sin(phi1 - phi2)) / sin(phi3 - phi2);
    j12 = (l1 * cos(phi0 - phi3) * sin(phi1 - phi2)) / (l0 * sin(phi3 - phi2));
    j21 = (l4 * sin(phi0 - phi2) * sin(phi3 - phi4)) / sin(phi3 - phi2);
    j22 = (l4 * cos(phi0 - phi2) * sin(phi3 - phi4)) / (l0 * sin(phi3 - phi2));
    J = [j11 j12;
         j21 j22];
    torque = J * [F; Tp];
    T1_L = torque(1, 1);
    T2_L = torque(2, 1);

== matlab function wheel_leg_robot/wheel_leg/MATLAB Function5 ==
  data: F input; T1_R output; Tp input; phi1 input; phi4 input; T2_R output
function [T1_R, T2_R] = fcn(F, Tp, phi1, phi4)

    l1 = 0.15;
    l2 = 0.27;
    l3 = l2;
    l4 = l1;
    l5 = 0.15;
    Xb = l1 * cos(phi1);
    Yb = l1 * sin(phi1);
    Xd = l4 * cos(phi4) + l5;
    Yd = l4 * sin(phi4);
    lbd = sqrt((Xd - Xb)^2 + (Yd - Yb)^2);
    A0 = 2 * l2 * (Xd - Xb);
    B0 = 2 * l2 * (Yd - Yb);
    C0 = l2^2 + lbd^2 - l3^2;
    phi2 = 2 * atan2((B0 + sqrt(A0^2 + B0^2 - C0^2)), (A0 + C0));
    phi3 = atan2(Yb - Yd + l2 * sin(phi2), Xb - Xd + l2 * cos(phi2));
    Xc = Xb + l2 * cos(phi2);
    Yc = Yb + l2 * sin(phi2);
    l0 = sqrt((Xc - l5/2)^2 + Yc^2);
    phi0 = atan2(Yc, (Xc - l5/2));
    j11 = (l1 * sin(phi0 - phi3) * sin(phi1 - phi2)) / sin(phi3 - phi2);
    j12 = (l1 * cos(phi0 - phi3) * sin(phi1 - phi2)) / (l0 * sin(phi3 - phi2));
    j21 = (l4 * sin(phi0 - phi2) * sin(phi3 - phi4)) / sin(phi3 - phi2);
    j22 = (l4 * cos(phi0 - phi2) * sin(phi3 - phi4)) / (l0 * sin(phi3 - phi2));
    J = [j11 j12;
         j21 j22];
    torque = J * [F; Tp];
    T1_R = torque(1, 1);
    T2_R = torque(2, 1);
